simulink model "DaVinci_Simul_DK"  (R2023a)
settings: Solver=VariableStepAuto  StartTime=0.0  StopTime=inf  RelTol=1e-3  EnableMultiTasking=on
libraries: vrlib x7, DaVinci_Lib x1
settings Model: Creator=jorgemartins  LastModifiedBy=afons
settings SolverCC: AlgebraicLoopSolver=TrustRegion
settings DataIOCC: LimitDataPoints=on  ReturnWorkspaceOutputs=off
settings OptimizationCC: LifeSpan=inf
settings DebuggingCC: UnconnectedInputMsg=warning  UnconnectedOutputMsg=warning  UnconnectedLineMsg=warning  AllowSymbolicDim=off  SFUnexpectedBacktrackingDiag=warning  SFNoUnconditionalDefaultTransitionDiag=warning  SFExecutionAtInitializationDiag=none  ArithmeticOperatorsInVariantConditions=warning
settings ModelReferenceCC: EnableRefExpFcnMdlSchedulingChecks=on  PropagateSignalLabelsOutOfModel=off
settings SFSimCC: SimUseLocalCustomCode=off  CustomCodeUndefinedFunction=UseInterfaceOnly
settings RTWCC: RTWUseLocalCustomCode=off
settings CodeAppCC: StateflowObjectComments=on
settings GRTTargetCC: TargetLangStandard=C89/C90 (ANSI)
settings ConfigComp: CovMetricSettings=dw  CovSaveCumulativeToWorkspaceVar=on  CovSaveSingleToWorkspaceVar=on  CovExternalEMLEnable=off

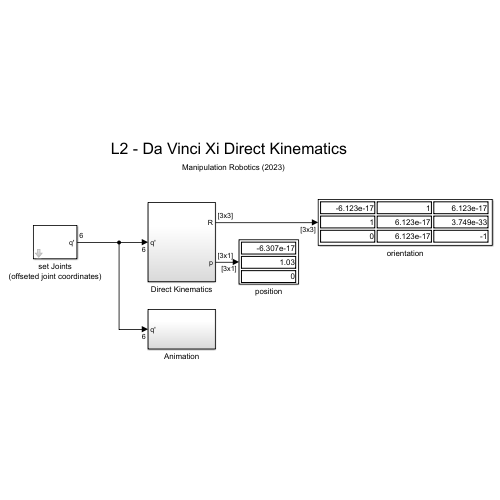
[thumbnail: Simulink's stored preview of the top-level diagram]
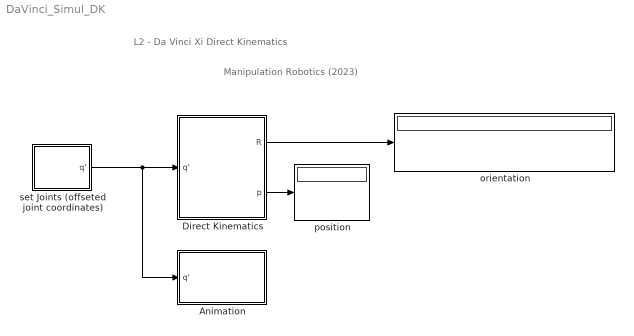
== system DaVinci_Simul_DK ==
  note: Manipulation Robotics (2023)
  note: L2 - Da Vinci Xi Direct Kinematics
  Animation : Subsystem
  Direct Kinematics : Subsystem
  orientation : Display
  position : Display
  set Joints (offseted joint coordinates) : Subsystem  mask{q1=-90, q2=0, q3=1, q4=90, q5=0, q6=0}
  wires:
  set Joints (offseted joint coordinates)/1(q') -> Animation/1(q'), Direct Kinematics/1(q')
  Direct Kinematics/1(R) -> orientation/1
  Direct Kinematics/2(p) -> position/1

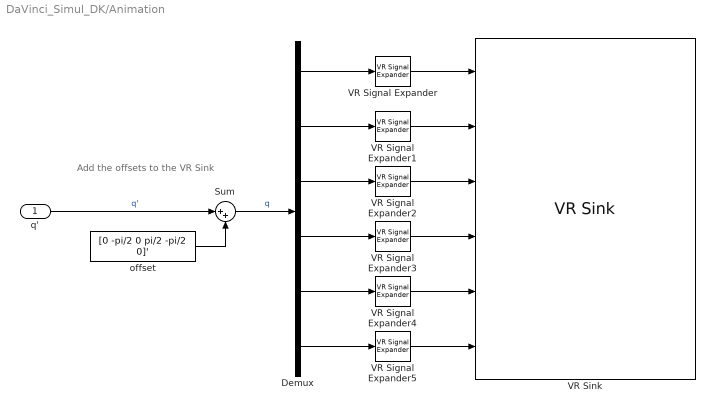
== system DaVinci_Simul_DK/Animation ==
  note: Add the offsets to the VR Sink
  q' : Inport
  Demux : Demux  Outputs=6
  Sum : Sum  Inputs=|++
  VR Signal Expander{,1,3..5} (5 alike) : vrlib/VR Signal Expander  outwidth=4  outidx=[4]
  VR Signal Expander2 : vrlib/VR Signal Expander  outwidth=3  outidx=[3]
  VR Sink : vrlib/VR Sink  InstantiateOnLoad=on  SampleTime=-1  ViewEnable=on  RemoteChange=off  RemoteView=off  FieldsWritten=Jt1_DH_dv.rotation.4.1.1.double#Jt2_DH_dv.rotation.4.1.1.double#Jt3_DH_dv.translation.3.1.1.double#Jt4_DH_dv.rotation.4.1.1.double#Jt5_DH_dv.rotation.4.1.1.double#Jt6_DH_dv.rotation.4.1.1.double  WorldFileName=DaVinciFrames.wrl  WorldDescription=Da Vinci Frames  AutoView=on  VideoDimensions=[]  AllowVariableSize=off  FigureProperties="{'Position', 'Name', 'Viewpoint', 'CameraBound', 'CameraDirection', 'CameraPosition', 'CameraUpVector', 'ZoomFactor', 'Antialiasing', 'Headlight', 'Lighting', 'NavPanel', 'Sound', 'StatusBar', 'Stereo3D', 'Stereo3DCameraOffset', 'Stereo3DHIT', 'ToolBar', 'Textures', 'Transparency', 'Triad', 'Wireframe', 'NavZones', 'NavMode', 'NavSpeed', 'CaptureFileFormat', 'CaptureFileName', 'Record2DCompressMethod', 'Record2DCompressQuality', 'Record2D', 'Record2DFileName', 'Record2DFPS'; [5.1539999999999998e+02   1.4059999999999991e+02   6.7919999999999993e+02   5.5560000000000002e+02], 'Da Vinci Frames', 'View 1', 'on', [-3.1811975811642412e-02   6.6406725291402027e-02   9.9728538795618804e-01], [-7.2925771628081934e-02  -1.1477675590687590e+00  -4.2021459022440801e+00], [9.5997266943557358e-01  -2.7577697323281780e-01   4.8985048445562125e-02], [1.0000000000000000e+00], 'on', 'on', 'on', 'halfbar', 'on', 'on', 'off', [1.0000000149011612e-01], [0.0000000000000000e+00], 'on', 'on', 'on', 'none', 'off', 'off', 'examine', 'normal', 'tif', '%f_anim_%n.tif', 'auto', [7.5000000000000000e+01], 'off', '%f_anim_%n.avi', 'auto'}"
  offset : Constant  Value=[0 -pi/2 0 pi/2 -pi/2 0]'  VectorParams1D=off
  wires:
  VR Signal Expander2/1 -> VR Sink/3
  offset/1 -> Sum/2
  VR Signal Expander1/1 -> VR Sink/2
  q'/1 -> Sum/1  "q'"
  Sum/1 -> Demux/1  "q"
  Demux/3 -> VR Signal Expander2/1
  Demux/6 -> VR Signal Expander5/1
  VR Signal Expander3/1 -> VR Sink/4
  Demux/1 -> VR Signal Expander/1
  Demux/2 -> VR Signal Expander1/1
  VR Signal Expander4/1 -> VR Sink/5
  Demux/4 -> VR Signal Expander3/1
  Demux/5 -> VR Signal Expander4/1
  VR Signal Expander5/1 -> VR Sink/6
  VR Signal Expander/1 -> VR Sink/1

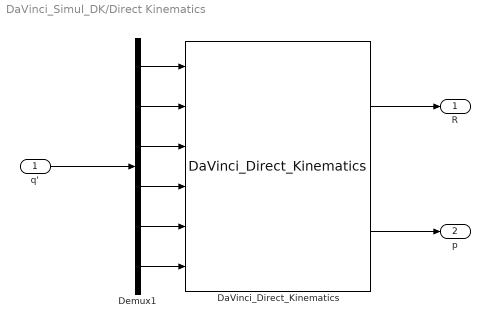
== system DaVinci_Simul_DK/Direct Kinematics ==
  q' : Inport
  DaVinci_Direct_Kinematics : DaVinci_Lib/DaVinci_Direct_Kinematics  SystemSampleTime=-1  VariantActivationTime=update diagram  Latency=0  AutoFrameSizeCalculation=off
  Demux1 : Demux  Outputs=6
  R : Outport
  p : Outport  Port=2
  wires:
  DaVinci_Direct_Kinematics/1 -> R/1
  DaVinci_Direct_Kinematics/2 -> p/1
  q'/1 -> Demux1/1
  Demux1/6 -> DaVinci_Direct_Kinematics/6
  Demux1/1 -> DaVinci_Direct_Kinematics/1
  Demux1/4 -> DaVinci_Direct_Kinematics/4
  Demux1/2 -> DaVinci_Direct_Kinematics/2
  Demux1/5 -> DaVinci_Direct_Kinematics/5
  Demux1/3 -> DaVinci_Direct_Kinematics/3

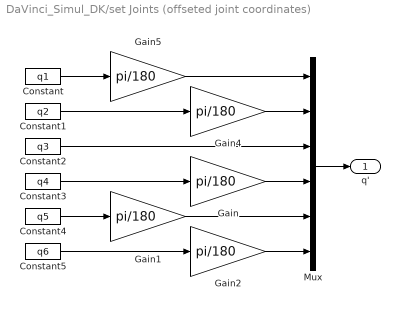
== system DaVinci_Simul_DK/set Joints (offseted joint coordinates) ==
  Constant : Constant  Value=q1
  Constant1 : Constant  Value=q2
  Constant2 : Constant  Value=q3
  Constant3 : Constant  Value=q4
  Constant4 : Constant  Value=q5
  Constant5 : Constant  Value=q6
  Gain{,1..2,4..5} (5 alike) : Gain  Gain=pi/180
  Mux : Mux  Inputs=6
  q' : Outport
  wires:
  Gain2/1 -> Mux/6
  Constant1/1 -> Gain4/1
  Constant3/1 -> Gain/1
  Constant5/1 -> Gain2/1
  Mux/1 -> q'/1
  Gain5/1 -> Mux/1
  Gain/1 -> Mux/4
  Gain1/1 -> Mux/5
  Gain4/1 -> Mux/2
  Constant/1 -> Gain5/1
  Constant2/1 -> Mux/3
  Constant4/1 -> Gain1/1
